simulink model "Model"  (R2023b)
settings: Solver=VariableStepAuto  StartTime=0.0  StopTime=40000  MaxStep=0.002  RelTol=1e-3
model workspace: external: MAT-File (data not in the file)
values from neighbouring files (symbols this model uses):
  CO =     [lambda_cp_my.mat]
  CO2 =     [lambda_cp_my.mat]
  Fe =     [lambda_cp_my.mat]
  Feox =     [lambda_cp_my.mat]
  H2 =     [lambda_cp_my.mat]
  H2O =     [lambda_cp_my.mat]
undefined symbols (not defined in the file or in its folder): var
settings Model: PacingRate=0.010000  Creator=A1201-admin  LastModifiedBy=A1201-admin
settings DataIOCC: LoadInitialState=on  SaveFinalState=on  SaveOperatingPoint=on

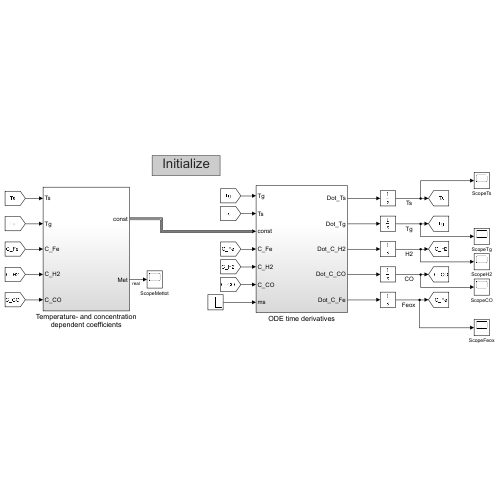
[thumbnail: Simulink's stored preview of the top-level diagram]
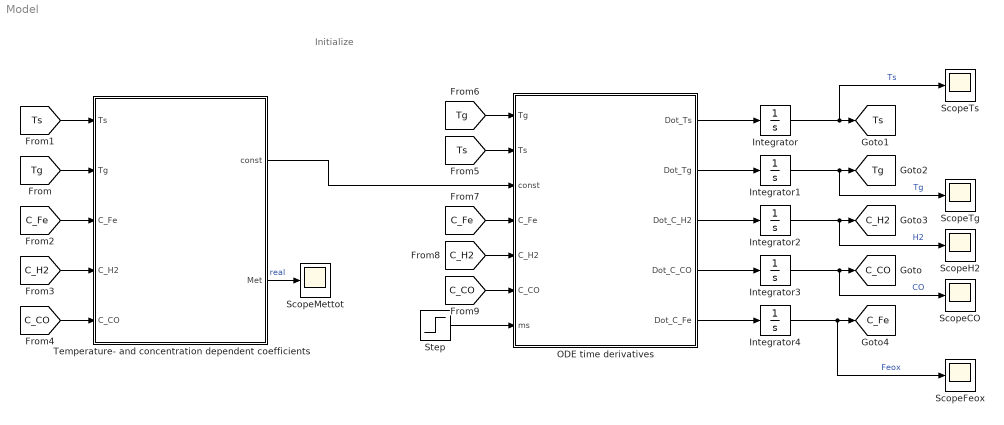
== system Model ==
  note: Initialize
  Integrator{,1..4} (5 alike) : Integrator
  ODE time derivatives : Subsystem
  ScopeCO : Scope
  ScopeFeox : Scope
  ScopeH2 : Scope
  ScopeMettot : Scope
  ScopeTg : Scope
  ScopeTs : Scope
  Step : Step  Time=500  Before=100  After=90  SampleTime=0
  Temperature- and concentration dependent coefficients : Subsystem
  tag scope: C_CO=global, C_Fe=global, C_H2=global, Tg=global, Ts=global
  wires:
  ODE time derivatives/4(Dot_C_CO) -> Integrator3/1
  ODE time derivatives/1(Dot_Ts) -> Integrator/1
  ODE time derivatives/2(Dot_Tg) -> Integrator1/1
  ODE time derivatives/3(Dot_C_H2) -> Integrator2/1
  ODE time derivatives/5(Dot_C_Fe) -> Integrator4/1
  Temperature- and concentration dependent coefficients/1(const) -> ODE time derivatives/3(const)
  [Tg] -> Temperature- and concentration dependent coefficients/2(Tg)
  [C_Fe] -> Temperature- and concentration dependent coefficients/3(C_Fe)
  [C_H2] -> Temperature- and concentration dependent coefficients/4(C_H2)
  [C_CO] -> Temperature- and concentration dependent coefficients/5(C_CO)
  [Ts] -> ODE time derivatives/2(Ts)
  [Tg] -> ODE time derivatives/1(Tg)
  [C_Fe] -> ODE time derivatives/4(C_Fe)
  [C_H2] -> ODE time derivatives/5(C_H2)
  [C_CO] -> ODE time derivatives/6(C_CO)
  Integrator/1 -> ScopeTs/1, [Ts]  "Ts"
  Integrator1/1 -> ScopeTg/1, [Tg]  "Tg"
  Integrator2/1 -> ScopeH2/1, [C_H2]  "H2"
  Integrator3/1 -> ScopeCO/1, [C_CO]  "CO"
  Integrator4/1 -> ScopeFeox/1, [C_Fe]  "Feox"
  [Ts] -> Temperature- and concentration dependent coefficients/1(Ts)
  Temperature- and concentration dependent coefficients/2(Met) -> ScopeMettot/1  "real"
  Step/1 -> ODE time derivatives/7(ms)

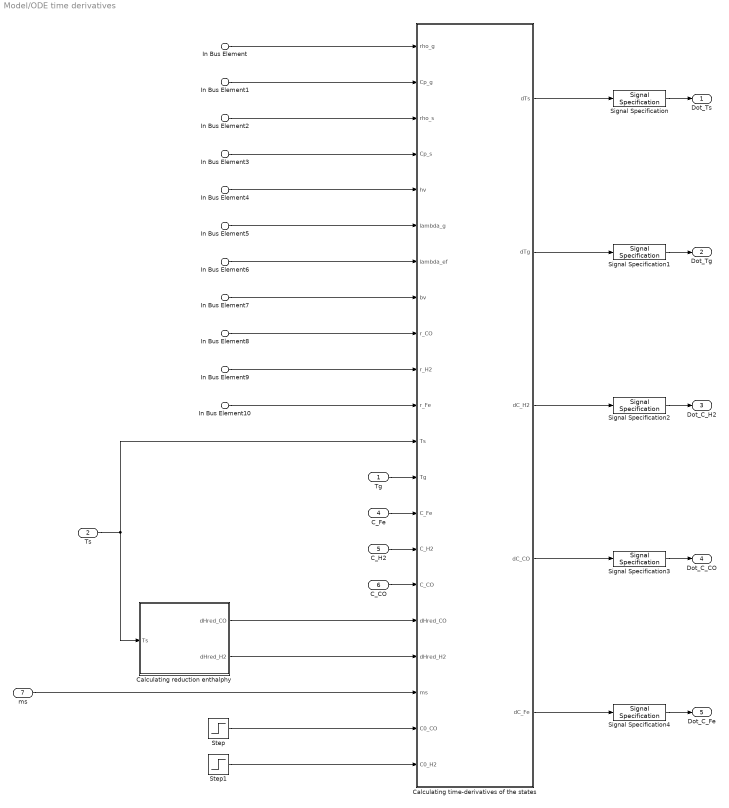
== system Model/ODE time derivatives ==
  Tg : Inport
  Ts : Inport  Port=2
  In Bus Element : Inport  Port=3  PortName=const  Element=rho_g
  In Bus Element1 : Inport  Port=3  PortName=const  Element=Cp_g
  In Bus Element2 : Inport  Port=3  PortName=const  Element=rho_s
  In Bus Element3 : Inport  Port=3  PortName=const  Element=Cp_s
  In Bus Element4 : Inport  Port=3  PortName=const  Element=hv
  In Bus Element5 : Inport  Port=3  PortName=const  Element=lambda_g
  In Bus Element6 : Inport  Port=3  PortName=const  Element=lambda_ef
  In Bus Element7 : Inport  Port=3  PortName=const  Element=bv
  In Bus Element8 : Inport  Port=3  PortName=const  Element=r_CO
  In Bus Element9 : Inport  Port=3  PortName=const  Element=r_H2
  In Bus Element10 : Inport  Port=3  PortName=const  Element=r_Fe
  C_Fe : Inport  Port=4
  C_H2 : Inport  Port=5
  C_CO : Inport  Port=6
  ms : Inport  Port=7
  Calculating reduction enthalphy : MATLAB Function  TreatAsAtomicUnit=on
  Calculating time-derivatives of the states : MATLAB Function  TreatAsAtomicUnit=on
  Signal Specification{,1..4} (5 alike) : SignalSpecification  Dimensions=[var.N,1]
  Step : Step  Time=500  Before=var.C0_CO  After=var.C0_CO  SampleTime=0
  Step1 : Step  Time=500  Before=var.C0_H2  After=2.2859  SampleTime=0
  Dot_Ts : Outport
  Dot_Tg : Outport  Port=2
  Dot_C_H2 : Outport  Port=3
  Dot_C_CO : Outport  Port=4
  Dot_C_Fe : Outport  Port=5
  wires:
  Ts/1 -> Calculating reduction enthalphy/1(Ts), Calculating time-derivatives of the states/12(Ts)
  In Bus Element/1 -> Calculating time-derivatives of the states/1(rho_g)
  Calculating time-derivatives of the states/3(dC_H2) -> Signal Specification2/1
  In Bus Element4/1 -> Calculating time-derivatives of the states/5(hv)
  In Bus Element7/1 -> Calculating time-derivatives of the states/8(bv)
  In Bus Element1/1 -> Calculating time-derivatives of the states/2(Cp_g)
  In Bus Element3/1 -> Calculating time-derivatives of the states/4(Cp_s)
  In Bus Element2/1 -> Calculating time-derivatives of the states/3(rho_s)
  In Bus Element5/1 -> Calculating time-derivatives of the states/6(lambda_g)
  Step1/1 -> Calculating time-derivatives of the states/21(C0_H2)
  In Bus Element6/1 -> Calculating time-derivatives of the states/7(lambda_ef)
  In Bus Element8/1 -> Calculating time-derivatives of the states/9(r_CO)
  In Bus Element9/1 -> Calculating time-derivatives of the states/10(r_H2)
  In Bus Element10/1 -> Calculating time-derivatives of the states/11(r_Fe)
  Tg/1 -> Calculating time-derivatives of the states/13(Tg)
  ms/1 -> Calculating time-derivatives of the states/19(ms)
  C_Fe/1 -> Calculating time-derivatives of the states/14(C_Fe)
  Signal Specification3/1 -> Dot_C_CO/1
  Calculating time-derivatives of the states/2(dTg) -> Signal Specification1/1
  C_H2/1 -> Calculating time-derivatives of the states/15(C_H2)
  Calculating time-derivatives of the states/4(dC_CO) -> Signal Specification3/1
  C_CO/1 -> Calculating time-derivatives of the states/16(C_CO)
  Calculating reduction enthalphy/1(dHred_CO) -> Calculating time-derivatives of the states/17(dHred_CO)
  Calculating reduction enthalphy/2(dHred_H2) -> Calculating time-derivatives of the states/18(dHred_H2)
  Step/1 -> Calculating time-derivatives of the states/20(C0_CO)
  Calculating time-derivatives of the states/1(dTs) -> Signal Specification/1
  Calculating time-derivatives of the states/5(dC_Fe) -> Signal Specification4/1
  Signal Specification/1 -> Dot_Ts/1
  Signal Specification1/1 -> Dot_Tg/1
  Signal Specification2/1 -> Dot_C_H2/1
  Signal Specification4/1 -> Dot_C_Fe/1

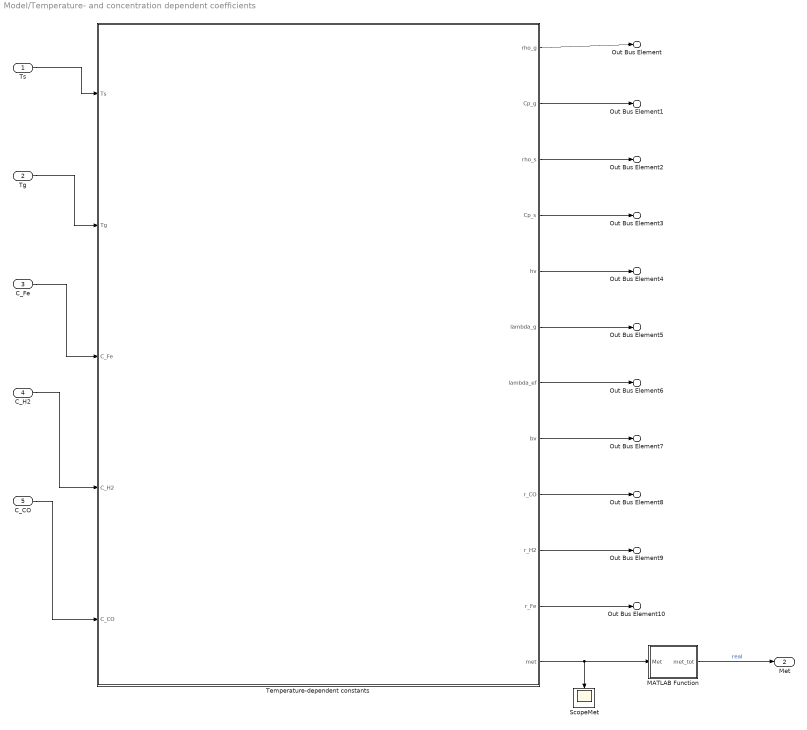
== system Model/Temperature- and concentration dependent coefficients ==
  Ts : Inport
  Tg : Inport  Port=2
  C_Fe : Inport  Port=3
  C_H2 : Inport  Port=4
  C_CO : Inport  Port=5
  MATLAB Function : MATLAB Function  TreatAsAtomicUnit=on
  ScopeMet : Scope
  Temperature-dependent constants : MATLAB Function  TreatAsAtomicUnit=on
  Out Bus Element : Outport  PortName=const  Element=rho_g
  Out Bus Element1 : Outport  PortName=const  Element=Cp_g
  Out Bus Element2 : Outport  PortName=const  Element=rho_s
  Out Bus Element3 : Outport  PortName=const  Element=Cp_s
  Out Bus Element4 : Outport  PortName=const  Element=hv
  Out Bus Element5 : Outport  PortName=const  Element=lambda_g
  Out Bus Element6 : Outport  PortName=const  Element=lambda_ef
  Out Bus Element7 : Outport  PortName=const  Element=bv
  Out Bus Element8 : Outport  PortName=const  Element=r_CO
  Out Bus Element9 : Outport  PortName=const  Element=r_H2
  Out Bus Element10 : Outport  PortName=const  Element=r_Fe
  Met : Outport  Port=2
  wires:
  C_CO/1 -> Temperature-dependent constants/5(C_CO)
  C_H2/1 -> Temperature-dependent constants/4(C_H2)
  C_Fe/1 -> Temperature-dependent constants/3(C_Fe)
  Tg/1 -> Temperature-dependent constants/2(Tg)
  Ts/1 -> Temperature-dependent constants/1(Ts)
  Temperature-dependent constants/6(lambda_g) -> Out Bus Element5/1
  Temperature-dependent constants/1(rho_g) -> Out Bus Element/1
  Temperature-dependent constants/2(Cp_g) -> Out Bus Element1/1
  Temperature-dependent constants/3(rho_s) -> Out Bus Element2/1
  Temperature-dependent constants/4(Cp_s) -> Out Bus Element3/1
  Temperature-dependent constants/5(hv) -> Out Bus Element4/1
  Temperature-dependent constants/7(lambda_ef) -> Out Bus Element6/1
  Temperature-dependent constants/8(bv) -> Out Bus Element7/1
  Temperature-dependent constants/9(r_CO) -> Out Bus Element8/1
  Temperature-dependent constants/10(r_H2) -> Out Bus Element9/1
  Temperature-dependent constants/11(r_Fe) -> Out Bus Element10/1
  Temperature-dependent constants/12(met) -> MATLAB Function/1(Met), ScopeMet/1
  MATLAB Function/1(met_tot) -> Met/1  "real"

== matlab function Model/ODE time derivatives/Calculating time-derivatives of the states ==
  settings: updateMethod=DISCRETE
  data: rho_g input; dTs output; Cp_g input; rho_s input; Cp_s input; hv input; lambda_g input; lambda_ef input; bv input; r_CO input; r_H2 input; r_Fe input; dTg output; dC_H2 output; dC_CO output; dC_Fe output; Ts input; Tg input; C_Fe input; C_H2 input; C_CO input; dHred_CO input; dHred_H2 input; var parameter; ms input; Fe parameter; C0_CO input; C0_H2 input
function [dTs,dTg, dC_H2, dC_CO, dC_Fe] = fcn(rho_g, Cp_g, rho_s, Cp_s,...
    hv, lambda_g, lambda_ef, bv, r_CO, r_H2, r_Fe, Ts, Tg, C_Fe, C_H2, C_CO...
    ,dHred_CO,dHred_H2,var,ms,Fe,C0_CO,C0_H2)

% This function block calculates the time derivative values of temperature
% and concentration, for all inner nodes and end-nodes.

Qvv = var.Qv*abs(r_Fe)*var.np;

%%%% Expressions if experiments with step changes are used %%%%

us =  ((ms/3.6)/(4*pi*(var.D/2)^3/3*Fe.rho))/var.np/(pi*(var.Dr/2)^2);
%us = var.us;
Tg0 = var.Tg0;
%C0_H2 = var.C0_H2/var.P*P;
%C0_CO = var.C0_CO/var.P*P;
%C0_H2 = var.C0_H2*var.Tg0/Tg0;
%C0_CO = var.C0_CO*var.Tg0/Tg0;
%C0_H2 = var.C0_H2;
%C0_CO = var.C0_CO;

%ug = var.ug*(var.P/(P));
ug = var.ug;
%ug = var.ug*Tg0/var.Tg0;



%%%%%%%%%%% Expressing time derivative of concentrations %%%%%%%%%%%%%%%%%%
% For Hydrogen

A_H2 = diag(-1*ones(var.N-1,1),-1) + diag(ones(var.N,1),0);
A_H2 = (-ug/(var.dz)).*A_H2;

b_H2 = var.np.*r_H2;
b_H2(1) = b_H2(1)-C0_H2*(-ug/(var.dz));

dC_H2 = A_H2*C_H2 + b_H2;

% For Carbon monoxide

A_CO = diag(-1*ones(var.N-1,1),-1) + diag(ones(var.N,1),0);
A_CO = (-ug/(var.dz)).*A_CO;

b_CO = var.np.*r_CO;
b_CO(1)= b_CO(1) - C0_CO*(-ug/(var.dz));

dC_CO = A_CO*C_CO + b_CO;

% For Iron 

A_Fe = diag(-1*ones(var.N,1),0) + diag(ones(var.N-1,1),1);
A_Fe = (us/(var.dz)).*A_Fe;

b_Fe = var.np.*r_Fe;
b_Fe(end) = b_Fe(end) + var.CL_Fe*(us/(var.dz));

dC_Fe = A_Fe*C_Fe + b_Fe;



%%%%%%%%%%%%% Upwind differencing %%%%%%%%%%%%%%%%%% https://www.etakl.net/notes_etc/numerical/schemes.pdf
%k = 1;
% Uncomment k and the expressions below "weighted with central diff" to try
% different weighings between unwind diff and central diff.


% Gas temperature

Kg1 = (var.e.*Cp_g.*rho_g.*ug)./var.dz + (var.e*lambda_g)./var.dz^2;
Kg2 = (-2*var.e*lambda_g)./var.dz^2 - hv - (var.e.*Cp_g.*rho_g*ug)./var.dz;
Kg3 = (var.e*lambda_g)./var.dz^2;

% Weighted with central diff
% Kg1 = (var.e.*Cp_g.*rho_g.*ug*(1+k))./(2*var.dz) + (var.e*lambda_g)./var.dz^2;
% Kg2 = (-2*var.e*lambda_g)./var.dz^2 - hv - (var.e.*Cp_g.*rho_g*ug*k)./var.dz;
% Kg3 = (var.e*lambda_g)./var.dz^2 - (var.e.*Cp_g.*rho_g*ug*(1-k))./(2*var.dz) ;


A_g = [(diag(Kg1(2:end),-1) + diag(Kg2,0) + diag(Kg3(1:end-1),1)),diag(hv)];


TgL = 2*Tg(end) - Tg(end-1);
b_g = [Qvv(1) + Kg1(1)*Tg0; Qvv(2:end-1); Qvv(end) + Kg3(end)*TgL];

dTg = (A_g*[Tg; Ts(1:end)] + b_g)./(var.e*Cp_g.*rho_g);


% Solid temperature

Ks1 = lambda_ef./var.dz^2;
Ks2 = (-2*lambda_ef./var.dz^2 - hv - bv - (Cp_s.*rho_s.*us*(1-var.e))./var.dz);
Ks3 = (lambda_ef)./var.dz^2 + (Cp_s.*rho_s*us*(1-var.e))/var.dz;
Ks4 = (1-var.e)*var.np*(dHred_CO.*r_CO + dHred_H2.*r_H2) + bv*var.T0;

% Weighted with central diff
% Ks1 = lambda_ef./var.dz^2 - (Cp_s.*rho_s.*us*(1-var.e)*(1-k))./(2*var.dz);
% Ks2 = (-2*lambda_ef./var.dz^2 - hv - bv - (Cp_s.*rho_s.*us*(1-var.e)*k)./var.dz);
% Ks3 = (lambda_ef)./var.dz^2 + (Cp_s.*rho_s*us*(1-var.e)*(1+k))/(2*var.dz);
% Ks4 = (1-var.e)*var.np*(dHred_CO.*r_CO + dHred_H2.*r_H2) + bv*var.T0;


A_s = [(diag(Ks1(2:end),-1) + diag(Ks2,0) + diag(Ks3(1:end-1),1)),diag(hv)];

Ts0 = 2*Ts(1) - Ts(2);
b_s = [Ks4(1) + Ks1(1)*Ts0 ;Ks4(2:end-1); Ks4(end) + Ks3(end)*var.TsL];

dTs = (A_s*[Ts; Tg(1:end)] + b_s)./((1-var.e)*Cp_s.*rho_s);



















end

== matlab function Model/ODE time derivatives/Calculating reduction enthalphy ==
  settings: updateMethod=DISCRETE
  data: dHred_CO output; dHred_H2 output; Ts input; H2 parameter; CO parameter; H2O parameter; CO2 parameter; Fe parameter; Feox parameter
function [dHred_CO, dHred_H2] = fcn(Ts, H2, CO, H2O, CO2, Fe, Feox)

% Calulates the reduction enthalpy for all reactions, based on the temperature-
% intergral of the specific heat capacity of the materials


CPint_H2 = interp1(H2.T,H2.CPint,Ts,'linear','extrap');
CPint_H2O = interp1(H2O.T,H2O.CPint,Ts,'linear','extrap');
CPint_CO = interp1(CO.T,CO.CPint,Ts,'linear','extrap');
CPint_CO2 = interp1(CO2.T,CO2.CPint,Ts,'linear','extrap');
CPint_Fe = interp1(Fe.T,Fe.CPint,Ts,'linear','extrap');
CPint_Feox = interp1(Feox.T,Feox.CPint,Ts,'linear','extrap');



dHred_CO = 2/3*(Fe.Hf0 + CPint_Fe) + (CO2.Hf0 + CPint_CO2) - 1/3*(Feox.Hf0 + CPint_Feox) - (CO.Hf0 + CPint_CO);


dHred_H2 = 2/3*(Fe.Hf0 + CPint_Fe) + (H2O.Hf0 + CPint_H2O) - 1/3*(Feox.Hf0 + CPint_Feox) - (H2.Hf0 + CPint_H2);




end

== matlab function Model/Temperature- and concentration dependent coefficients/Temperature-dependent constants ==
  settings: updateMethod=DISCRETE
  data: Ts input; Tg input; rho_g output; Cp_g output; rho_s output; Cp_s output; hv output; lambda_g output; lambda_ef output; bv output; r_CO output; r_H2 output; r_Fe output; C_Fe input; C_H2 input; C_CO input; CO parameter; Fe parameter; Feox parameter; H2 parameter; var parameter; met output
function [rho_g,Cp_g,rho_s,Cp_s,hv,lambda_g,lambda_ef,bv,r_CO,r_H2,r_Fe,met]...
         = fcn(Ts, Tg, C_Fe, C_H2, C_CO, CO, Fe, Feox, H2, var)
 
% This function block calculates all necessary coefficients used in the 
% time-derivatives, based on thermal and concentration dependent material
% parameters.

%%%%%%%%%% Interpolate from tabulated values %%%%%%%%%%%%%%
CP_Fe = mean(interp1(Fe.T,Fe.CP,Ts,'linear','extrap'));
CP_Feox = mean(interp1(Feox.T,Feox.CP,Ts,'linear','extrap'));
lambda_Feox = mean(interp1(Feox.T,Feox.lambda,Ts,'linear','extrap'));
lambda_Fe = mean(interp1(Fe.T,Fe.lambda,Ts,'linear','extrap'));
lambda_CO = mean(interp1(CO.T,CO.lambda,Tg,'linear','extrap'));
lambda_H2 = mean(interp1(H2.T,H2.lambda,Tg,'linear','extrap'));
my_CO = mean(interp1(CO.T,CO.my,Tg,'linear','extrap'));
my_H2 = mean(interp1(H2.T,H2.my,Tg,'linear','extrap'));
CP_CO = mean(interp1(CO.T,CO.CP,Tg,'linear','extrap'));
CP_H2 = mean(interp1(H2.T,H2.CP,Tg,'linear','extrap'));

%ug = var.ug*(var.P/(P));

%ug = var.ug*Tg0/var.Tg0;

ug = var.ug ;
%%%%%%%%%%% Gas Constants  %%%%%%%%%%%%%%%%%%%%

    x_co = C_CO./(C_CO+C_H2); % fraction = Ci/Ctot
    x_h2 = C_H2./(C_CO+C_H2);

    Mg = x_co.*CO.M + x_h2.*H2.M; % = sum of fraction*molecular weight

    Cp_g = x_co.*CP_CO + x_h2.*CP_H2; % = sum of fraction*CP  

    phi_h2co = (1 + (my_H2./my_CO).^0.5*(CO.M/H2.M)^0.25).^2./(8*(1+H2.M/CO.M))^0.5;

    phi_coh2 = (1 + (my_CO./my_H2).^0.5*(H2.M/CO.M)^0.25).^2./(8*(1+CO.M/H2.M))^0.5;

    my_g = x_h2.*my_H2./(x_h2+x_co.*phi_h2co) + x_co.*my_CO./(x_h2.*phi_coh2+x_co);

    lambda_g = x_h2.*lambda_H2./(x_h2+x_co.*phi_h2co) + x_co.*lambda_CO./(x_h2.*phi_coh2+x_co);

    rho_g = var.P*Mg./(var.Ru*Tg);%/var.P*P; % Palacios

   
%%%%%%%%%%%%%%%%%%%%%%%% Solid constants %%%%%%%%%%%%%%%%%%%%%%%%%%%%%%%%%%
    Co = 3*(var.CL_Fe - C_Fe); % Palacios

    rc = ((var.D/2)^3 - Co*Feox.M/(var.np*4*pi*Feox.rho)).^(1/3); % Palacios

    Cp_s = (CP_Feox.*Feox.rho.*rc.^3 + CP_Fe.*Fe.rho.*((var.D/2)^3-rc.^3))./...
    (Feox.rho*rc.^3 + Fe.rho*((var.D/2)^3-rc.^3)); % Palacios

    lambda_s = (lambda_Feox.*Feox.rho.*rc.^3 + lambda_Fe.*Fe.rho.*((var.D/2)^3-rc.^3))./...
    (Feox.rho.*rc.^3 + Fe.rho.*((var.D/2)^3-rc.^3)); % Palacios
    
    rho_s = (Feox.rho*rc.^3+Fe.rho*((var.D/2)^3-rc.^3))/(var.D/2)^3; % Palacios


%%%%%%%%%%%%%%%%%%%%%% Heat transfer Coeff %%%%%%%%%%%%%%%%%%%%%%%%%%%%%%%%    
    Pr = my_g.*Cp_g./lambda_g; % By definition

    %Re = var.D*var.e*ug*rho_g./((1-var.e)*my_g); % perrys chemical engineers handbook

    Re = var.D*var.e*ug*rho_g./(my_g); % Heat and mass transfer in packed beds

    Nu = 2 + 1.1*Pr.^(1/3).*Re.^(0.6); % Palacios

    hv = 6*(1-var.e)*lambda_g.*Nu/var.D^2; % Palacios

    lambda_ef = 0.005*lambda_s+4*5.67051e-8*var.D*Ts.^3*(var.e/(1-var.e)); % Palacios
    
    bv = 4/var.Dc*(var.h+var.emiss_s*var.trans_r*5.67051e-8*(Ts.^4 - var.T0^4)./(Ts-var.T0)); % Palacios
  

%%%%%%%%%%%%%%%%%%%%%%%% Kinetics Coeff %%%%%%%%%%%%%%%%%%%%%%%%%%%%%%%%%%% 
    
    
    
    Ap = 4*pi*(var.D/2)^2; % Palacios
    
    k_h2 = 0.00225*exp(-14700./(82.06*Ts)); %From Parisi via Palacios

    k_co = 0.0065*exp(-28100./(82.06*Ts)); %From Parisi via Palacios

    De_h2 = 1.467e-10*Ts.^(1.75); %From Parisi via Palacios

    De_co = 3.828e-11*Ts.^(1.75); %From Parisi via Palacios

    r_CO = -C_CO*var.zeta*Ap./(1./k_co + (var.D/2)*((var.D/2)-rc)./(rc.*De_co) + (var.D/2)^2./(rc.^2.*k_co)); % Palacios
    
    r_H2 = -C_H2*var.xi*Ap./(1./k_h2 + (var.D/2)*((var.D/2)-rc)./(rc.*De_h2) + (var.D/2)^2./(rc.^2.*k_h2)); % Palacios
    
    r_Fe = var.b*(r_H2+r_CO); % Palacios
    
    met = Co./(3*var.CL_Fe);
    

end

== matlab function Model/Temperature- and concentration dependent coefficients/MATLAB Function ==
  data: Met input; met_tot output
function met_tot = fcn(Met)

met_tot = 2*Met(1) - Met(2);
